simulink model "FCS_MPC_6ph_testbench_single_test"  (R2022a)
settings: Solver=ode23t  StartTime=0.0  StopTime=0.1  RelTol=1e-3  AbsTol=1e-3  EnableMultiTasking=on
values from neighbouring files (symbols this model uses):
  f_c = 100000    [Params_testbench.m]
  L_d = 0.0001473    [Params_testbench.m]
  L_q = 0.0001484    [Params_testbench.m]
  L_x = 0.00005566    (= 5.566e-05)    [Params_testbench.m]
  L_y = L_x    (= 5.566e-05)    [Params_testbench.m]
  p = 5    [Params_testbench.m]
  psi_pm = 0.0048    [Params_testbench.m]
  R_ph = 0.1278    [Params_testbench.m]
  u_dc = 36.0    (= 36)    [Params_testbench.m]
libraries: nesl_utility x39, fl_lib x32, hdlsllib x26, ee_lib x12, simulink x2, spsAlphaBetaZerotodq0Lib x1
(part 4 of 4)

== matlab function FCS_MPC_6ph_testbench_single_test/Microcontroller Software/Prediction_and_cost_function/Subsystem/MATLAB Function10 ==
  data: SampleTime_div_Ld input; J output; SampleTime_div_Lq input; SampleTime_div_Lx input; SampleTime_div_Ly input; id_k_1 input; iq_k_1 input; ix_k_1 input; iy_k_1 input; Rs input; omega_el input; Lq input; Ld input; psiPM input; d_phase_voltage_per_switching_state input; q_phase_voltage_per_switching_state input; x_phase_voltage_per_switching_state input; y_phase_voltage_per_switching_state input; id_ref input; iq_ref input; ix_ref input; iy_ref input
function J = fcn(SampleTime_div_Ld, SampleTime_div_Lq, SampleTime_div_Lx, SampleTime_div_Ly, id_k_1, iq_k_1, ix_k_1, iy_k_1, Rs, omega_el, Lq, Ld, psiPM, d_phase_voltage_per_switching_state, q_phase_voltage_per_switching_state, x_phase_voltage_per_switching_state, y_phase_voltage_per_switching_state, id_ref, iq_ref, ix_ref, iy_ref)
     
        % Prediction of the d-, q-, x-, y-currents of the 6-Phase-PMSM with the finite control set 
        id_k_2 = single(SampleTime_div_Ld*(d_phase_voltage_per_switching_state-id_k_1*Rs+omega_el*Lq*iq_k_1)+id_k_1);
        iq_k_2 = single(SampleTime_div_Lq*(q_phase_voltage_per_switching_state-iq_k_1*Rs-omega_el*(psiPM+id_k_1*Ld))+iq_k_1);
        ix_k_2 = single(SampleTime_div_Lx*(x_phase_voltage_per_switching_state-ix_k_1*Rs)+ix_k_1);
        iy_k_2 = single(SampleTime_div_Ly*(y_phase_voltage_per_switching_state-iy_k_1*Rs)+iy_k_1);
        
        % Calculation of the cost function
        J = single((id_ref-id_k_2)^2+(iq_ref-iq_k_2)^2+(ix_ref-ix_k_2)^2+(iy_ref-iy_k_2)^2);

end

== matlab function FCS_MPC_6ph_testbench_single_test/Microcontroller Software/Prediction_and_cost_function/Subsystem/MATLAB Function11 ==
  data: SampleTime_div_Ld input; J output; SampleTime_div_Lq input; SampleTime_div_Lx input; SampleTime_div_Ly input; id_k_1 input; iq_k_1 input; ix_k_1 input; iy_k_1 input; Rs input; omega_el input; Lq input; Ld input; psiPM input; d_phase_voltage_per_switching_state input; q_phase_voltage_per_switching_state input; x_phase_voltage_per_switching_state input; y_phase_voltage_per_switching_state input; id_ref input; iq_ref input; ix_ref input; iy_ref input
function J = fcn(SampleTime_div_Ld, SampleTime_div_Lq, SampleTime_div_Lx, SampleTime_div_Ly, id_k_1, iq_k_1, ix_k_1, iy_k_1, Rs, omega_el, Lq, Ld, psiPM, d_phase_voltage_per_switching_state, q_phase_voltage_per_switching_state, x_phase_voltage_per_switching_state, y_phase_voltage_per_switching_state, id_ref, iq_ref, ix_ref, iy_ref)
     
        % Prediction of the d-, q-, x-, y-currents of the 6-Phase-PMSM with the finite control set 
        id_k_2 = single(SampleTime_div_Ld*(d_phase_voltage_per_switching_state-id_k_1*Rs+omega_el*Lq*iq_k_1)+id_k_1);
        iq_k_2 = single(SampleTime_div_Lq*(q_phase_voltage_per_switching_state-iq_k_1*Rs-omega_el*(psiPM+id_k_1*Ld))+iq_k_1);
        ix_k_2 = single(SampleTime_div_Lx*(x_phase_voltage_per_switching_state-ix_k_1*Rs)+ix_k_1);
        iy_k_2 = single(SampleTime_div_Ly*(y_phase_voltage_per_switching_state-iy_k_1*Rs)+iy_k_1);
        
        % Calculation of the cost function
        J = single((id_ref-id_k_2)^2+(iq_ref-iq_k_2)^2+(ix_ref-ix_k_2)^2+(iy_ref-iy_k_2)^2);

end

== matlab function FCS_MPC_6ph_testbench_single_test/Microcontroller Software/Prediction_and_cost_function/Subsystem/MATLAB Function12 ==
  data: SampleTime_div_Ld input; J output; SampleTime_div_Lq input; SampleTime_div_Lx input; SampleTime_div_Ly input; id_k_1 input; iq_k_1 input; ix_k_1 input; iy_k_1 input; Rs input; omega_el input; Lq input; Ld input; psiPM input; d_phase_voltage_per_switching_state input; q_phase_voltage_per_switching_state input; x_phase_voltage_per_switching_state input; y_phase_voltage_per_switching_state input; id_ref input; iq_ref input; ix_ref input; iy_ref input
function J = fcn(SampleTime_div_Ld, SampleTime_div_Lq, SampleTime_div_Lx, SampleTime_div_Ly, id_k_1, iq_k_1, ix_k_1, iy_k_1, Rs, omega_el, Lq, Ld, psiPM, d_phase_voltage_per_switching_state, q_phase_voltage_per_switching_state, x_phase_voltage_per_switching_state, y_phase_voltage_per_switching_state, id_ref, iq_ref, ix_ref, iy_ref)
     
        % Prediction of the d-, q-, x-, y-currents of the 6-Phase-PMSM with the finite control set 
        id_k_2 = single(SampleTime_div_Ld*(d_phase_voltage_per_switching_state-id_k_1*Rs+omega_el*Lq*iq_k_1)+id_k_1);
        iq_k_2 = single(SampleTime_div_Lq*(q_phase_voltage_per_switching_state-iq_k_1*Rs-omega_el*(psiPM+id_k_1*Ld))+iq_k_1);
        ix_k_2 = single(SampleTime_div_Lx*(x_phase_voltage_per_switching_state-ix_k_1*Rs)+ix_k_1);
        iy_k_2 = single(SampleTime_div_Ly*(y_phase_voltage_per_switching_state-iy_k_1*Rs)+iy_k_1);
        
        % Calculation of the cost function
        J = single((id_ref-id_k_2)^2+(iq_ref-iq_k_2)^2+(ix_ref-ix_k_2)^2+(iy_ref-iy_k_2)^2);

end

== matlab function FCS_MPC_6ph_testbench_single_test/Microcontroller Software/Prediction_and_cost_function/Subsystem/MATLAB Function13 ==
  data: SampleTime_div_Ld input; J output; SampleTime_div_Lq input; SampleTime_div_Lx input; SampleTime_div_Ly input; id_k_1 input; iq_k_1 input; ix_k_1 input; iy_k_1 input; Rs input; omega_el input; Lq input; Ld input; psiPM input; d_phase_voltage_per_switching_state input; q_phase_voltage_per_switching_state input; x_phase_voltage_per_switching_state input; y_phase_voltage_per_switching_state input; id_ref input; iq_ref input; ix_ref input; iy_ref input
function J = fcn(SampleTime_div_Ld, SampleTime_div_Lq, SampleTime_div_Lx, SampleTime_div_Ly, id_k_1, iq_k_1, ix_k_1, iy_k_1, Rs, omega_el, Lq, Ld, psiPM, d_phase_voltage_per_switching_state, q_phase_voltage_per_switching_state, x_phase_voltage_per_switching_state, y_phase_voltage_per_switching_state, id_ref, iq_ref, ix_ref, iy_ref)
     
        % Prediction of the d-, q-, x-, y-currents of the 6-Phase-PMSM with the finite control set 
        id_k_2 = single(SampleTime_div_Ld*(d_phase_voltage_per_switching_state-id_k_1*Rs+omega_el*Lq*iq_k_1)+id_k_1);
        iq_k_2 = single(SampleTime_div_Lq*(q_phase_voltage_per_switching_state-iq_k_1*Rs-omega_el*(psiPM+id_k_1*Ld))+iq_k_1);
        ix_k_2 = single(SampleTime_div_Lx*(x_phase_voltage_per_switching_state-ix_k_1*Rs)+ix_k_1);
        iy_k_2 = single(SampleTime_div_Ly*(y_phase_voltage_per_switching_state-iy_k_1*Rs)+iy_k_1);
        
        % Calculation of the cost function
        J = single((id_ref-id_k_2)^2+(iq_ref-iq_k_2)^2+(ix_ref-ix_k_2)^2+(iy_ref-iy_k_2)^2);

end

== matlab function FCS_MPC_6ph_testbench_single_test/Microcontroller Software/Prediction_and_cost_function/Subsystem/MATLAB Function14 ==
  data: SampleTime_div_Ld input; J output; SampleTime_div_Lq input; SampleTime_div_Lx input; SampleTime_div_Ly input; id_k_1 input; iq_k_1 input; ix_k_1 input; iy_k_1 input; Rs input; omega_el input; Lq input; Ld input; psiPM input; d_phase_voltage_per_switching_state input; q_phase_voltage_per_switching_state input; x_phase_voltage_per_switching_state input; y_phase_voltage_per_switching_state input; id_ref input; iq_ref input; ix_ref input; iy_ref input
function J = fcn(SampleTime_div_Ld, SampleTime_div_Lq, SampleTime_div_Lx, SampleTime_div_Ly, id_k_1, iq_k_1, ix_k_1, iy_k_1, Rs, omega_el, Lq, Ld, psiPM, d_phase_voltage_per_switching_state, q_phase_voltage_per_switching_state, x_phase_voltage_per_switching_state, y_phase_voltage_per_switching_state, id_ref, iq_ref, ix_ref, iy_ref)
     
        % Prediction of the d-, q-, x-, y-currents of the 6-Phase-PMSM with the finite control set 
        id_k_2 = single(SampleTime_div_Ld*(d_phase_voltage_per_switching_state-id_k_1*Rs+omega_el*Lq*iq_k_1)+id_k_1);
        iq_k_2 = single(SampleTime_div_Lq*(q_phase_voltage_per_switching_state-iq_k_1*Rs-omega_el*(psiPM+id_k_1*Ld))+iq_k_1);
        ix_k_2 = single(SampleTime_div_Lx*(x_phase_voltage_per_switching_state-ix_k_1*Rs)+ix_k_1);
        iy_k_2 = single(SampleTime_div_Ly*(y_phase_voltage_per_switching_state-iy_k_1*Rs)+iy_k_1);
        
        % Calculation of the cost function
        J = single((id_ref-id_k_2)^2+(iq_ref-iq_k_2)^2+(ix_ref-ix_k_2)^2+(iy_ref-iy_k_2)^2);
      

end

== matlab function FCS_MPC_6ph_testbench_single_test/Microcontroller Software/Prediction_and_cost_function/Subsystem/MATLAB Function15 ==
  data: SampleTime_div_Ld input; J output; SampleTime_div_Lq input; SampleTime_div_Lx input; SampleTime_div_Ly input; id_k_1 input; iq_k_1 input; ix_k_1 input; iy_k_1 input; Rs input; omega_el input; Lq input; Ld input; psiPM input; d_phase_voltage_per_switching_state input; q_phase_voltage_per_switching_state input; x_phase_voltage_per_switching_state input; y_phase_voltage_per_switching_state input; id_ref input; iq_ref input; ix_ref input; iy_ref input
function J = fcn(SampleTime_div_Ld, SampleTime_div_Lq, SampleTime_div_Lx, SampleTime_div_Ly, id_k_1, iq_k_1, ix_k_1, iy_k_1, Rs, omega_el, Lq, Ld, psiPM, d_phase_voltage_per_switching_state, q_phase_voltage_per_switching_state, x_phase_voltage_per_switching_state, y_phase_voltage_per_switching_state, id_ref, iq_ref, ix_ref, iy_ref)
     
        % Prediction of the d-, q-, x-, y-currents of the 6-Phase-PMSM with the finite control set 
        id_k_2 = single(SampleTime_div_Ld*(d_phase_voltage_per_switching_state-id_k_1*Rs+omega_el*Lq*iq_k_1)+id_k_1);
        iq_k_2 = single(SampleTime_div_Lq*(q_phase_voltage_per_switching_state-iq_k_1*Rs-omega_el*(psiPM+id_k_1*Ld))+iq_k_1);
        ix_k_2 = single(SampleTime_div_Lx*(x_phase_voltage_per_switching_state-ix_k_1*Rs)+ix_k_1);
        iy_k_2 = single(SampleTime_div_Ly*(y_phase_voltage_per_switching_state-iy_k_1*Rs)+iy_k_1);
        
        % Calculation of the cost function
        J = single((id_ref-id_k_2)^2+(iq_ref-iq_k_2)^2+(ix_ref-ix_k_2)^2+(iy_ref-iy_k_2)^2);

end

== matlab function FCS_MPC_6ph_testbench_single_test/Microcontroller Software/Min_cost_function_and_vopt2/MATLAB Function ==
  data: J_1 input; Index_1 input int32; voltages_1 input; J_2 input; Index_2 input int32; voltages_2 input; J_3 input; Index_3 input int32; voltages_3 input; J_4 input; Index_4 input int32; voltages_4 input; J_5 input; Index_5 input int32; voltages_5 input; J_6 input; Index_6 input int32; voltages_6 input; J_7 input; Index_7 input int32; voltages_7 input; J_8 input; Index_8 input int32; voltages_8 input; Index output int32; voltages output; min input; voltages_default input
function [Index, voltages] = fcn(J_1, Index_1, voltages_1, J_2, Index_2, voltages_2, J_3, Index_3, voltages_3, J_4, Index_4, voltages_4, J_5, Index_5, voltages_5, J_6, Index_6, voltages_6, ...
                                    J_7, Index_7, voltages_7, J_8, Index_8, voltages_8, min,voltages_default)



if J_1 == min
    Index = Index_1;
    voltages = voltages_1;
elseif J_2 == min
    Index = Index_2;
    voltages = voltages_2;
elseif J_3 == min
    Index = Index_3;
    voltages = voltages_3;
elseif J_4 == min
    Index = Index_4;
    voltages = voltages_4;
elseif J_5 == min
    Index = Index_5;
    voltages = voltages_5;
elseif J_6 == min
    Index = Index_6;
    voltages = voltages_6;
elseif J_7 == min
    Index = Index_7;
    voltages = voltages_7;
elseif J_8 == min
    Index = Index_8;
    voltages = voltages_8;
else 
    Index = int32(0);
    voltages = voltages_default;
end

== matlab function FCS_MPC_6ph_testbench_single_test/Microcontroller Software/Phase_voltages_per_switching_state2/Subsystem/MATLAB Function10 ==
  data: sin_theta_el input; cos_theta_el input; d_voltage_per_switching_state output; u_dc_link_voltage input; Index input; q_voltage_per_switching_state output; x_voltage_per_switching_state output; y_voltage_per_switching_state output
function [d_voltage_per_switching_state, q_voltage_per_switching_state, x_voltage_per_switching_state, y_voltage_per_switching_state] = fcn(sin_theta_el, cos_theta_el, u_dc_link_voltage, Index)
      
        % Initial condition
            Index = Index+1;

        % Swichtingstates factors alpha beta x y
        Factors_alpha_beta_x_y = single([0.288675134594813	 0.622008467928146	 0.122008467928146	 0.455341801261480    0.122008467928146	 0.455341801261480	-0.0446581987385205  0.288675134594813;
                                         -0.166666666666667	-0.166666666666667	 0.122008467928146	 0.122008467928146   -0.455341801261480	-0.455341801261480	-0.166666666666667	-0.166666666666667;
                                         -0.288675134594813	 0.0446581987385205	-0.455341801261480	-0.122008467928146   -0.455341801261480	-0.122008467928146	-0.622008467928146	-0.288675134594813;
                                         -0.166666666666667	-0.166666666666667	-0.455341801261480	-0.455341801261480    0.122008467928146	 0.122008467928146	-0.166666666666667	-0.166666666666667]);
        
        % Park-Transformation of the switchingstates factors
        Factors_d_q_x_y =single(zeros(4,1));
    
        Factors_d_q_x_y(3,1) = Factors_alpha_beta_x_y(3,Index);
        Factors_d_q_x_y(4,1) = Factors_alpha_beta_x_y(4,Index);
       
        Factors_d_q_x_y(1,1) = cos_theta_el*Factors_alpha_beta_x_y(1,Index)+sin_theta_el*Factors_alpha_beta_x_y(2,Index);
        Factors_d_q_x_y(2,1) = -sin_theta_el*Factors_alpha_beta_x_y(1,Index)+cos_theta_el*Factors_alpha_beta_x_y(2,Index);
    
        %Calculation of the voltages per switching state in alpha beta coordinates
        d_q_x_y_voltages_per_switching_state = single(u_dc_link_voltage*Factors_d_q_x_y);
    
        d_voltage_per_switching_state = d_q_x_y_voltages_per_switching_state(1,1);
        q_voltage_per_switching_state = d_q_x_y_voltages_per_switching_state(2,1);
        x_voltage_per_switching_state = d_q_x_y_voltages_per_switching_state(3,1);
        y_voltage_per_switching_state = d_q_x_y_voltages_per_switching_state(4,1);
    

end

== matlab function FCS_MPC_6ph_testbench_single_test/Microcontroller Software/Phase_voltages_per_switching_state2/Subsystem/MATLAB Function11 ==
  data: sin_theta_el input; cos_theta_el input; d_voltage_per_switching_state output; u_dc_link_voltage input; Index input; q_voltage_per_switching_state output; x_voltage_per_switching_state output; y_voltage_per_switching_state output
function [d_voltage_per_switching_state, q_voltage_per_switching_state, x_voltage_per_switching_state, y_voltage_per_switching_state] = fcn(sin_theta_el, cos_theta_el, u_dc_link_voltage, Index)
      
        % Initial condition
            Index = Index+1;

    
        % Swichtingstates factors alpha beta x y
        Factors_alpha_beta_x_y = single([0	                 0.333333333333333	-0.166666666666667	  0.166666666666667    -0.166666666666667	  0.166666666666667	    -0.333333333333333	 0;
                                        -0.333333333333333	-0.333333333333333	-0.0446581987385205	 -0.0446581987385205   -0.622008467928146	 -0.622008467928146	    -0.333333333333333	-0.333333333333333;
                                         0	                 0.333333333333333	-0.166666666666667	  0.166666666666667    -0.166666666666667	  0.166666666666667	    -0.333333333333333	 0;
                                        -0.333333333333333	-0.333333333333333	-0.622008467928146	 -0.622008467928146    -0.0446581987385205   -0.0446581987385205	-0.333333333333333	-0.333333333333333]);
        
        % Park-Transformation of the switchingstates factors
        Factors_d_q_x_y =single(zeros(4,1));
    
        Factors_d_q_x_y(3,1) = Factors_alpha_beta_x_y(3,Index);
        Factors_d_q_x_y(4,1) = Factors_alpha_beta_x_y(4,Index);

        Factors_d_q_x_y(1,1) = cos_theta_el*Factors_alpha_beta_x_y(1,Index)+sin_theta_el*Factors_alpha_beta_x_y(2,Index);
        Factors_d_q_x_y(2,1) = -sin_theta_el*Factors_alpha_beta_x_y(1,Index)+cos_theta_el*Factors_alpha_beta_x_y(2,Index);
    
        %Calculation of the voltages per switching state in alpha beta coordinates
        d_q_x_y_voltages_per_switching_state = single(u_dc_link_voltage*Factors_d_q_x_y);
    
        d_voltage_per_switching_state = d_q_x_y_voltages_per_switching_state(1,1);
        q_voltage_per_switching_state = d_q_x_y_voltages_per_switching_state(2,1);
        x_voltage_per_switching_state = d_q_x_y_voltages_per_switching_state(3,1);
        y_voltage_per_switching_state = d_q_x_y_voltages_per_switching_state(4,1);
    

end

== matlab function FCS_MPC_6ph_testbench_single_test/Microcontroller Software/Phase_voltages_per_switching_state2/Subsystem/MATLAB Function12 ==
  data: sin_theta_el input; cos_theta_el input; d_voltage_per_switching_state output; u_dc_link_voltage input; Index input; q_voltage_per_switching_state output; x_voltage_per_switching_state output; y_voltage_per_switching_state output
function [d_voltage_per_switching_state, q_voltage_per_switching_state, x_voltage_per_switching_state, y_voltage_per_switching_state] = fcn(sin_theta_el, cos_theta_el, u_dc_link_voltage, Index)
      
        % Initial condition
            Index = Index+1;

    
        % Swichtingstates factors alpha beta x y
        Factors_alpha_beta_x_y = single([0	                0.333333333333333	-0.166666666666667  	0.166666666666667   -0.166666666666667	 0.166666666666667	 -0.333333333333333	0;
                                         0.333333333333333	0.333333333333333	 0.622008467928146	    0.622008467928146    0.0446581987385205	 0.0446581987385205	  0.333333333333333	0.333333333333333;
                                         0	                0.333333333333333	-0.166666666666667	    0.166666666666667   -0.166666666666667	 0.166666666666667	 -0.333333333333333	0;
                                         0.333333333333333	0.333333333333333	 0.0446581987385205 	0.0446581987385205   0.622008467928146	 0.622008467928146	  0.333333333333333	0.333333333333333]);
        
        % Park-Transformation of the switchingstates factors
        Factors_d_q_x_y =single(zeros(4,1));
    
        Factors_d_q_x_y(3,1) = Factors_alpha_beta_x_y(3,Index);
        Factors_d_q_x_y(4,1) = Factors_alpha_beta_x_y(4,Index);
           
        Factors_d_q_x_y(1,1) = cos_theta_el*Factors_alpha_beta_x_y(1,Index)+sin_theta_el*Factors_alpha_beta_x_y(2,Index);
        Factors_d_q_x_y(2,1) = -sin_theta_el*Factors_alpha_beta_x_y(1,Index)+cos_theta_el*Factors_alpha_beta_x_y(2,Index);
    
        %Calculation of the voltages per switching state in alpha beta coordinates
        d_q_x_y_voltages_per_switching_state = single(u_dc_link_voltage*Factors_d_q_x_y);
    
        d_voltage_per_switching_state = d_q_x_y_voltages_per_switching_state(1,1);
        q_voltage_per_switching_state = d_q_x_y_voltages_per_switching_state(2,1);
        x_voltage_per_switching_state = d_q_x_y_voltages_per_switching_state(3,1);
        y_voltage_per_switching_state = d_q_x_y_voltages_per_switching_state(4,1);
    

end

== matlab function FCS_MPC_6ph_testbench_single_test/Microcontroller Software/Phase_voltages_per_switching_state2/Subsystem/MATLAB Function13 ==
  data: sin_theta_el input; cos_theta_el input; d_voltage_per_switching_state output; u_dc_link_voltage input; Index input; q_voltage_per_switching_state output; x_voltage_per_switching_state output; y_voltage_per_switching_state output
function [d_voltage_per_switching_state, q_voltage_per_switching_state, x_voltage_per_switching_state, y_voltage_per_switching_state] = fcn(sin_theta_el, cos_theta_el, u_dc_link_voltage, Index)
      
        % Initial condition
            Index = Index+1;

    
        % Swichtingstates factors alpha beta x y
        Factors_alpha_beta_x_y = single([-0.288675134594813	0.0446581987385205	-0.455341801261480	-0.122008467928146   -0.455341801261480	-0.122008467928146	-0.622008467928146	-0.288675134594813;
                                         0.166666666666667	0.166666666666667	 0.455341801261480   0.455341801261480   -0.122008467928146	-0.122008467928146	 0.166666666666667	 0.166666666666667;
                                         0.288675134594813	0.622008467928146	 0.122008467928146	 0.455341801261480    0.122008467928146	 0.455341801261480	-0.0446581987385205	 0.288675134594813;
                                         0.166666666666667	0.166666666666667	-0.122008467928146	-0.122008467928146    0.455341801261480	 0.455341801261480	 0.166666666666667	 0.166666666666667]);
        
        % Park-Transformation of the switchingstates factors
        Factors_d_q_x_y =single(zeros(4,1));
    
        Factors_d_q_x_y(3,1) = Factors_alpha_beta_x_y(3,Index);
        Factors_d_q_x_y(4,1) = Factors_alpha_beta_x_y(4,Index);
           
        Factors_d_q_x_y(1,1) = cos_theta_el*Factors_alpha_beta_x_y(1,Index)+sin_theta_el*Factors_alpha_beta_x_y(2,Index);
        Factors_d_q_x_y(2,1) = -sin_theta_el*Factors_alpha_beta_x_y(1,Index)+cos_theta_el*Factors_alpha_beta_x_y(2,Index);
    
        %Calculation of the voltages per switching state in alpha beta coordinates
        d_q_x_y_voltages_per_switching_state = single(u_dc_link_voltage*Factors_d_q_x_y);
    
        d_voltage_per_switching_state = d_q_x_y_voltages_per_switching_state(1,1);
        q_voltage_per_switching_state = d_q_x_y_voltages_per_switching_state(2,1);
        x_voltage_per_switching_state = d_q_x_y_voltages_per_switching_state(3,1);
        y_voltage_per_switching_state = d_q_x_y_voltages_per_switching_state(4,1);
    

end

== matlab function FCS_MPC_6ph_testbench_single_test/Microcontroller Software/Phase_voltages_per_switching_state2/Subsystem/MATLAB Function14 ==
  data: sin_theta_el input; cos_theta_el input; d_voltage_per_switching_state output; u_dc_link_voltage input; Index input; q_voltage_per_switching_state output; x_voltage_per_switching_state output; y_voltage_per_switching_state output
function [d_voltage_per_switching_state, q_voltage_per_switching_state, x_voltage_per_switching_state, y_voltage_per_switching_state] = fcn(sin_theta_el, cos_theta_el, u_dc_link_voltage, Index)
      
        % Initial condition
            Index = Index+1;

    
        % Swichtingstates factors alpha beta x y
        Factors_alpha_beta_x_y = single([0.288675134594813	0.622008467928146	 0.122008467928146  	0.455341801261480     0.122008467928146	 0.455341801261480	-0.0446581987385205  0.288675134594813;   
                                         0.166666666666667	0.166666666666667	 0.455341801261480  	0.455341801261480    -0.122008467928146	-0.122008467928146	 0.166666666666667	 0.166666666666667;
                                         -0.288675134594813	0.0446581987385205	-0.455341801261480	   -0.122008467928146    -0.455341801261480	-0.122008467928146	-0.622008467928146	-0.288675134594813;
                                         0.166666666666667	0.166666666666667	-0.122008467928146     -0.122008467928146     0.455341801261480	 0.455341801261480	 0.166666666666667	 0.166666666666667]);
        
        % Park-Transformation of the switchingstates factors
        Factors_d_q_x_y =single(zeros(4,1));
    
        Factors_d_q_x_y(3,1) = Factors_alpha_beta_x_y(3,Index);
        Factors_d_q_x_y(4,1) = Factors_alpha_beta_x_y(4,Index);
       
        Factors_d_q_x_y(1,1) = cos_theta_el*Factors_alpha_beta_x_y(1,Index)+sin_theta_el*Factors_alpha_beta_x_y(2,Index);
        Factors_d_q_x_y(2,1) = -sin_theta_el*Factors_alpha_beta_x_y(1,Index)+cos_theta_el*Factors_alpha_beta_x_y(2,Index);
    
        %Calculation of the voltages per switching state in alpha beta coordinates
        d_q_x_y_voltages_per_switching_state = single(u_dc_link_voltage*Factors_d_q_x_y);
    
        d_voltage_per_switching_state = d_q_x_y_voltages_per_switching_state(1,1);
        q_voltage_per_switching_state = d_q_x_y_voltages_per_switching_state(2,1);
        x_voltage_per_switching_state = d_q_x_y_voltages_per_switching_state(3,1);
        y_voltage_per_switching_state = d_q_x_y_voltages_per_switching_state(4,1);
    

end

== matlab function FCS_MPC_6ph_testbench_single_test/Microcontroller Software/Phase_voltages_per_switching_state2/Subsystem/MATLAB Function15 ==
  data: sin_theta_el input; cos_theta_el input; d_voltage_per_switching_state output; u_dc_link_voltage input; Index input; q_voltage_per_switching_state output; x_voltage_per_switching_state output; y_voltage_per_switching_state output
function [d_voltage_per_switching_state, q_voltage_per_switching_state, x_voltage_per_switching_state, y_voltage_per_switching_state] = fcn(sin_theta_el, cos_theta_el, u_dc_link_voltage, Index)
      
        % Initial condition
            Index = Index+1;

        % Swichtingstates factors alpha beta x y
        Factors_alpha_beta_x_y = single([0	    0.333333333333333	-0.166666666666667	 0.166666666666667    -0.166666666666667	 0.166666666666667	-0.333333333333333	0;
                                         0	    0                    0.288675134594813	 0.288675134594813    -0.288675134594813	-0.288675134594813	 0	                0;
                                         0	    0.333333333333333	-0.166666666666667	 0.166666666666667    -0.166666666666667	 0.166666666666667	-0.333333333333333	0;
                                         0	    0	                -0.288675134594813	-0.288675134594813     0.288675134594813	 0.288675134594813	 0              	0]);
        
        % Park-Transformation of the switchingstates factors
        Factors_d_q_x_y =single(zeros(4,1));
    
        Factors_d_q_x_y(3,1) = Factors_alpha_beta_x_y(3,Index);
        Factors_d_q_x_y(4,1) = Factors_alpha_beta_x_y(4,Index);
          
        Factors_d_q_x_y(1,1) = cos_theta_el*Factors_alpha_beta_x_y(1,Index)+sin_theta_el*Factors_alpha_beta_x_y(2,Index);
        Factors_d_q_x_y(2,1) = -sin_theta_el*Factors_alpha_beta_x_y(1,Index)+cos_theta_el*Factors_alpha_beta_x_y(2,Index);
    
        %Calculation of the voltages per switching state in alpha beta coordinates
        d_q_x_y_voltages_per_switching_state = single(u_dc_link_voltage*Factors_d_q_x_y);
    
        d_voltage_per_switching_state = d_q_x_y_voltages_per_switching_state(1,1);
        q_voltage_per_switching_state = d_q_x_y_voltages_per_switching_state(2,1);
        x_voltage_per_switching_state = d_q_x_y_voltages_per_switching_state(3,1);
        y_voltage_per_switching_state = d_q_x_y_voltages_per_switching_state(4,1);
    

end

== matlab function FCS_MPC_6ph_testbench_single_test/Microcontroller Software/Phase_voltages_per_switching_state2/Subsystem/MATLAB Function8 ==
  data: sin_theta_el input; cos_theta_el input; d_voltage_per_switching_state output; u_dc_link_voltage input; Index input; q_voltage_per_switching_state output; x_voltage_per_switching_state output; y_voltage_per_switching_state output
function [d_voltage_per_switching_state, q_voltage_per_switching_state, x_voltage_per_switching_state, y_voltage_per_switching_state] = fcn(sin_theta_el, cos_theta_el, u_dc_link_voltage, Index)
      
        % Initial condition
            Index = Index+1;

    
        % Swichtingstates factors alpha beta x y
        Factors_alpha_beta_x_y = single([0	0.333333333333333	-0.166666666666667	 0.166666666666667    -0.166666666666667	 0.166666666666667	-0.333333333333333	0;
                                         0	0	                 0.288675134594813	 0.288675134594813    -0.288675134594813	-0.288675134594813	 0	                0;
                                         0	0.333333333333333	-0.166666666666667	 0.166666666666667    -0.166666666666667	 0.166666666666667	-0.333333333333333	0;
                                         0	0	                -0.288675134594813	-0.288675134594813     0.288675134594813	 0.288675134594813	 0	                0]);
        
        % Park-Transformation of the switchingstates factors
        Factors_d_q_x_y =single(zeros(4,1));
    
        Factors_d_q_x_y(3,1) = Factors_alpha_beta_x_y(3,Index);
        Factors_d_q_x_y(4,1) = Factors_alpha_beta_x_y(4,Index);
       
        Factors_d_q_x_y(1,1) = cos_theta_el*Factors_alpha_beta_x_y(1,Index)+sin_theta_el*Factors_alpha_beta_x_y(2,Index);
        Factors_d_q_x_y(2,1) = -sin_theta_el*Factors_alpha_beta_x_y(1,Index)+cos_theta_el*Factors_alpha_beta_x_y(2,Index);
    
        %Calculation of the voltages per switching state in alpha beta coordinates
        d_q_x_y_voltages_per_switching_state = single(u_dc_link_voltage*Factors_d_q_x_y);
    
        d_voltage_per_switching_state = d_q_x_y_voltages_per_switching_state(1,1);
        q_voltage_per_switching_state = d_q_x_y_voltages_per_switching_state(2,1);
        x_voltage_per_switching_state = d_q_x_y_voltages_per_switching_state(3,1);
        y_voltage_per_switching_state = d_q_x_y_voltages_per_switching_state(4,1);
    

end

== matlab function FCS_MPC_6ph_testbench_single_test/Microcontroller Software/Phase_voltages_per_switching_state2/Subsystem/MATLAB Function9 ==
  data: sin_theta_el input; cos_theta_el input; d_voltage_per_switching_state output; u_dc_link_voltage input; Index input; q_voltage_per_switching_state output; x_voltage_per_switching_state output; y_voltage_per_switching_state output
function [d_voltage_per_switching_state, q_voltage_per_switching_state, x_voltage_per_switching_state, y_voltage_per_switching_state] = fcn(sin_theta_el, cos_theta_el, u_dc_link_voltage, Index)
      
        % Initial condition
            Index = Index+1;

    
        % Swichtingstates factors alpha beta x y
        Factors_alpha_beta_x_y = single([-0.288675134594813	 0.0446581987385205  -0.455341801261480	  -0.122008467928146    -0.455341801261480	-0.122008467928146	-0.622008467928146	-0.288675134594813;
                                         -0.166666666666667	-0.166666666666667	  0.122008467928146	   0.122008467928146    -0.455341801261480	-0.455341801261480	-0.166666666666667	-0.166666666666667;
                                         0.288675134594813	 0.622008467928146	  0.122008467928146	   0.455341801261480     0.122008467928146	 0.455341801261480	-0.0446581987385205  0.288675134594813;
                                         -0.166666666666667	-0.166666666666667	 -0.455341801261480	  -0.455341801261480     0.122008467928146	 0.122008467928146	-0.166666666666667	-0.166666666666667]);
        
        % Park-Transformation of the switchingstates factors
        Factors_d_q_x_y =single(zeros(4,1));
    
        Factors_d_q_x_y(3,1) = Factors_alpha_beta_x_y(3,Index);
        Factors_d_q_x_y(4,1) = Factors_alpha_beta_x_y(4,Index);
       
        Factors_d_q_x_y(1,1) = cos_theta_el*Factors_alpha_beta_x_y(1,Index)+sin_theta_el*Factors_alpha_beta_x_y(2,Index);
        Factors_d_q_x_y(2,1) = -sin_theta_el*Factors_alpha_beta_x_y(1,Index)+cos_theta_el*Factors_alpha_beta_x_y(2,Index);
    
        %Calculation of the voltages per switching state in alpha beta coordinates
        d_q_x_y_voltages_per_switching_state = single(u_dc_link_voltage*Factors_d_q_x_y);
    
        d_voltage_per_switching_state = d_q_x_y_voltages_per_switching_state(1,1);
        q_voltage_per_switching_state = d_q_x_y_voltages_per_switching_state(2,1);
        x_voltage_per_switching_state = d_q_x_y_voltages_per_switching_state(3,1);
        y_voltage_per_switching_state = d_q_x_y_voltages_per_switching_state(4,1);
    

end

== matlab function FCS_MPC_6ph_testbench_single_test/Microcontroller Software/vsd_and_park_tra/MATLAB Function ==
  settings: fimath=fimath('RoundingMethod', 'Floor','OverflowAction', 'Wrap','ProductMode', 'FullPrecision', 'SumMode', 'FullPrecision')
  data: i_a1 input; i_alpha output; i_b1 input; i_c1 input; i_a2 input; i_b2 input; i_c2 input; sin_theta_el input; i_beta output; i_x output; i_y output; i_0_plus output; i_0_minus output; i_d output; i_q output; cos_theta_el input
function [i_alpha,i_beta,i_x,i_y,i_0_plus,i_0_minus,i_d,i_q] = VSD_and_Park_transformation(i_a1,i_b1,i_c1,i_a2,i_b2,i_c2,sin_theta_el,cos_theta_el)

    % VSD-Transformation
    A = [0 0 0 0 0 0]';

    A =  0.3333*[1    -0.5        -0.5        0.8660   -0.8660  0 ;
                0    0.8660   -0.8660  0.5         0.5         -1;
                1    -0.5        -0.5        -0.8660  0.8660   0 ;
                0    -0.8660  0.8660   0.5         0.5         -1;
                1    1           1           0           0           0 ;
                0    0           0           1           1           1] * [i_a1 i_b1 i_c1 i_a2 i_b2 i_c2]';

    i_alpha = A(1);
    i_beta = A(2);
    i_x = A(3);
    i_y = A(4);
    i_0_plus = A(5);
    i_0_minus = A(6);

    % Park-Transformation
%    B = [0 0]';

%     B = [cos(theta_el)       sin(theta_el);
%         -sin(theta_el)       cos(theta_el)] * [i_alpha i_beta]';

 %   i_d = B(1);
 %   i_q = B(2);



i_d = cos_theta_el*i_alpha+sin_theta_el*i_beta;
i_q = -sin_theta_el*i_alpha+cos_theta_el*i_beta;


end

== matlab function FCS_MPC_6ph_testbench_single_test/Microcontroller Software/Delay_compensation/MATLAB Function ==
  data: SampleTime_div_Ld input; SampleTime_div_Lq input; SampleTime_div_Lx input; SampleTime_div_Ly input; id_k_1 output; last_applied_optimal_voltage_d input; last_applied_optimal_voltage_q input; last_applied_optimal_voltage_x input; last_applied_optimal_voltage_y input; id_measured input; iq_measured input; ix_measured input; iy_measured input; psiPM input; Lq input; Ld input; Rs input; iq_k_1 output; ix_k_1 output; iy_k_1 output; omega_el input
function [id_k_1, iq_k_1, ix_k_1, iy_k_1] = fcn(SampleTime_div_Ld, SampleTime_div_Lq, SampleTime_div_Lx, SampleTime_div_Ly, last_applied_optimal_voltage_d, last_applied_optimal_voltage_q, last_applied_optimal_voltage_x, last_applied_optimal_voltage_y, id_measured, iq_measured, ix_measured, iy_measured, psiPM, Lq, Ld, Rs, omega_el)
  
    % Delay compensation with a modell of a 6-Phase PMSM
    id_k_1 = single(SampleTime_div_Ld*(last_applied_optimal_voltage_d-id_measured*Rs+omega_el*Lq*iq_measured)+id_measured);
    iq_k_1 = single(SampleTime_div_Lq*(last_applied_optimal_voltage_q-iq_measured*Rs-omega_el*(psiPM+id_measured*Ld))+iq_measured);
    ix_k_1 = single(SampleTime_div_Lx*(last_applied_optimal_voltage_x-ix_measured*Rs)+ix_measured);
    iy_k_1 = single(SampleTime_div_Ly*(last_applied_optimal_voltage_y-iy_measured*Rs)+iy_measured);

end
